simulink model "OpAmp_integrator"  (R2017a)
settings: Solver=VariableStepAuto  StartTime=0.0  StopTime=7  MaxStep=1e-3  RelTol=1e-3
libraries: fl_lib x5, elec_lib x4, nesl_utility x4
settings Model: Creator=erich  LastModifiedBy=erich

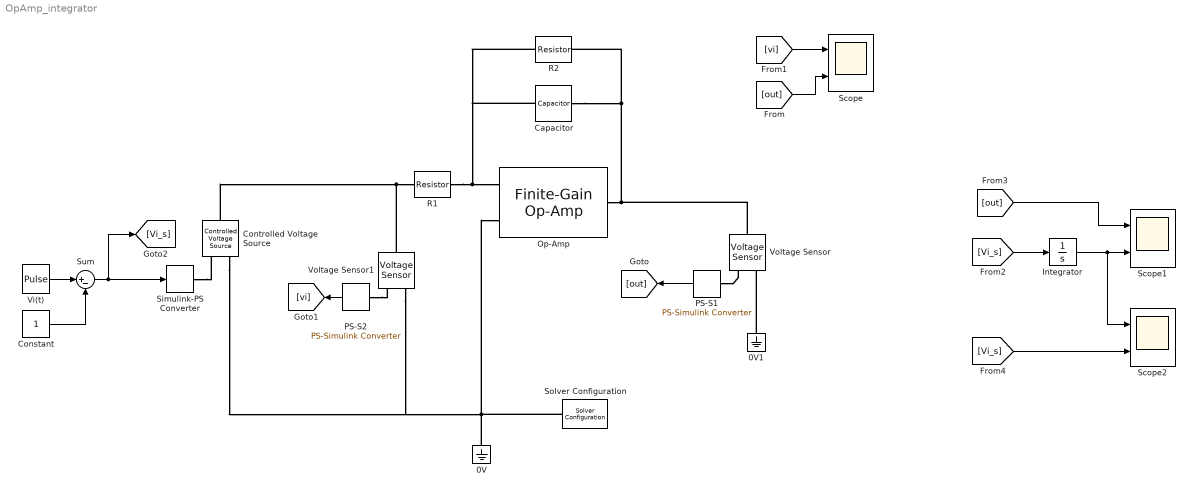
== system OpAmp_integrator ==
  0V : fl_lib/Electrical/Electrical Elements/Electrical Reference
  0V1 : fl_lib/Electrical/Electrical Elements/Electrical Reference
  Capacitor : elec_lib/Passive Devices/Capacitor  enable_table=0  c=220e-6 F  Cvec=[1.0e-5, 1.0e-6] F  Vvec=[0.0, 10.0] V  CV_table_symmetry=1  C_tol=5  enable_C_tol=0  tol_distribution=1  nSigma=4  r=1e-6 Ohm  g=0 1/Ohm  enable_operating_limits=0  operating_limit_action=2  max_working_voltage_range=[-25.0, 25.0] V  power_rating=1 W  enable_faults=0  fault_action=1  Cscale_faulted=100  R_faulted=1e-3 Ohm  G_faulted=0 1/Ohm  tau_fault=1e-3 s  enable_temporal_fault=0  t_fault=1 s  enable_behavioral_fault=0  max_permissible_voltage_range=[-100.0, 100.0] V  t_fail_on_voltage=1 s  i_specify=off  i_priority=None  i=0 A  i_nominal_specify=off  i_nominal_unit=A  i_nominal_value=1  v_specify=off  v_priority=None  v=0 V  v_nominal_specify=off  v_nominal_unit=V  v_nominal_value=1  vc_specify=off  vc_priority=High  vc=0 V  vc_nominal_specify=off  vc_nominal_unit=V  vc_nominal_value=1
  Constant : Constant
  Controlled Voltage Source : fl_lib/Electrical/Electrical Sources/Controlled Voltage Source
  Integrator : Integrator  InitialCondition=-.05
  Op-Amp : elec_lib/Integrated Circuits/Finite-Gain Op-Amp  A=2000  Rin=1e6 Ohm  Rout=100 Ohm  Vmin=-15 V  Vmax=15 V
      settings: SourceProductName=Simscape Electronics  SourceProductBaseCode=SN
  PS-S1 : nesl_utility/PS-Simulink Converter  PhysicalDomain=network_engine_domain  SubClassName=ps_output  LeftPortType=input  RightPortType=output  PseudoPeriodic=off  Frequencies=[]  Unit=1  AffineConversion=off
  PS-S2 : nesl_utility/PS-Simulink Converter  PhysicalDomain=network_engine_domain  SubClassName=ps_output  LeftPortType=input  RightPortType=output  PseudoPeriodic=off  Frequencies=[]  Unit=1  AffineConversion=off
  R1 : elec_lib/Passive Devices/Resistor  R=1 kOhm  R_tol=5  enable_R_tol=0  tol_distribution=1  nSigma=4  enable_operating_limits=0  operating_limit_action=2  max_working_voltage=100 V  power_rating=1 W  enable_faults=0  fault_action=1  R_faulted=inf Ohm  enable_temporal_fault=0  t_fault=1 s  enable_behavioral_fault=0  max_permissible_current=1 A  t_fail_on_current=1 s  noise_mode=0  sample_time=1e-3 s  repeatability=1  auto_seed=3046698749  user_seed=0  Tdevice=25 degC  alpha=3.93e-3 1/K  Tmeas=25 degC  thermal_mass=100 J/K  power_derating_T1=70 degC  power_derating_T2=155 degC  operating_temperature_range_vec=[-50.0, 150.0] degC  temperature_specify=off  temperature_priority=High  temperature=298.15 K  temperature_nominal_specify=off  temperature_nominal_unit=K  temperature_nominal_value=1
  R2 : elec_lib/Passive Devices/Resistor  R=1 kOhm  R_tol=5  enable_R_tol=0  tol_distribution=1  nSigma=4  enable_operating_limits=0  operating_limit_action=2  max_working_voltage=100 V  power_rating=1 W  enable_faults=0  fault_action=1  R_faulted=inf Ohm  enable_temporal_fault=0  t_fault=1 s  enable_behavioral_fault=0  max_permissible_current=1 A  t_fail_on_current=1 s  noise_mode=0  sample_time=1e-3 s  repeatability=1  auto_seed=4278366030  user_seed=0  Tdevice=25 degC  alpha=3.93e-3 1/K  Tmeas=25 degC  thermal_mass=100 J/K  power_derating_T1=70 degC  power_derating_T2=155 degC  operating_temperature_range_vec=[-50.0, 150.0] degC  temperature_specify=off  temperature_priority=High  temperature=298.15 K  temperature_nominal_specify=off  temperature_nominal_unit=K  temperature_nominal_value=1
  Scope : Scope  NumInputPorts=2
  Scope1 : Scope  NumInputPorts=2
  Scope2 : Scope  NumInputPorts=2
  Simulink-PS Converter : nesl_utility/Simulink-PS Converter  PhysicalDomain=network_engine_domain  SubClassName=ps_input  LeftPortType=input  RightPortType=output  PseudoPeriodic=off  Frequencies=[]  NoiseDistribution=none  NoiseParameters=[]  Unit=1  AffineConversion=off  FilteringAndDerivatives=provide  SimscapeFilterOrder=1  InputFilterTimeConstant=0.001  UdotUserProvided=0
  Solver Configuration : nesl_utility/Solver Configuration  PhysicalDomain=network_engine_domain  SubClassName=solver  LeftPortType=input  RightPortType=generic  Accelerate=off  Tones=[]  Harmonics=[]  SimulateNoise=off  Profile=off  UseLocalSampling=off  EnableSwitchedLinearOptims=on  FrequencyDomain=off  UseCCode=off  RelTol=0.001  AbsTol=1e-06  MinStep=1e-09  ToWorkspace=off  RevertToSquareIcSolve=off  NumHomotopyIterations=100  PhasorMode=off  PhasorModeNumHarmonics=1  OverrideAbsTol=off  DoDC=off  ResidualTolerance=1e-09  UseLocalSolver=off  LocalSolverChoice=NE_BACKWARD_EULER_ADVANCER  LocalSolverSampleTime=0.001  DoFixedCost=off  MaxNonlinIter=3  MaxModeIter=2  LinearAlgebra=Sparse  DelaysMemoryBudget=1024  AutomaticFiltering=on  FilteringTimeConstant=0.001
  Sum : Sum  Inputs=|+-
  Vi(t) : DiscretePulseGenerator  PulseType=Time based  Amplitude=2  Period=.2  PulseWidth=50
  Voltage Sensor : fl_lib/Electrical/Electrical Sensors/Voltage Sensor
  Voltage Sensor1 : fl_lib/Electrical/Electrical Sensors/Voltage Sensor
  wires:
  PS-S1/1 -> [out]
  [out] -> Scope/2
  PS-S2/1 -> [vi]
  [vi] -> Scope/1
  Sum/1 -> [Vi_s], Simulink-PS Converter/1
  Vi(t)/1 -> Sum/1
  Constant/1 -> Sum/2
  [Vi_s] -> Integrator/1
  Integrator/1 -> Scope2/1, Scope1/2
  [out] -> Scope1/1
  [Vi_s] -> Scope2/2
  connections:
  0V/LConn1 -- Solver Configuration/RConn1 -- Op-Amp/LConn1 -- Controlled Voltage Source/RConn2 -- Voltage Sensor1/RConn2
  R1/RConn1 -- Op-Amp/LConn2 -- Capacitor/LConn1 -- R2/LConn1
  Op-Amp/RConn1 -- Capacitor/RConn1 -- R2/RConn1 -- Voltage Sensor/LConn1
  0V1/LConn1 -- Voltage Sensor/RConn2
  PS-S1/LConn1 -- Voltage Sensor/RConn1
  Voltage Sensor1/LConn1 -- Controlled Voltage Source/LConn1 -- R1/LConn1
  Simulink-PS Converter/RConn1 -- Controlled Voltage Source/RConn1
  PS-S2/LConn1 -- Voltage Sensor1/RConn1
